simulink model "proj7_highway"  (R2016b)
settings: Solver=ode4  StartTime=0.0  StopTime=765  FixedStep=1  RelTol=1e-3  EnableMultiTasking=on
values from neighbouring files (symbols this model uses):
  V = sch_cycle(:,2)    [Motor_plot.m]
undefined symbols (not defined in the file or in its folder): mc
settings Model: Creator=dave0651  LastModifiedBy=Jinesh
settings OptimizationCC: LifeSpan=inf
settings DebuggingCC: SFUnexpectedBacktrackingDiag=warning  SFNoUnconditionalDefaultTransitionDiag=warning  SFExecutionAtInitializationDiag=none
settings GRTTargetCC: TargetLangStandard=C89/C90 (ANSI)  GeneratePreprocessorConditionals=Disable all
settings ConfigComp: CovMetricSettings=dw  CovHtmlReporting=on  CovSaveCumulativeToWorkspaceVar=on  CovSaveSingleToWorkspaceVar=on  CovExternalEMLEnable=off

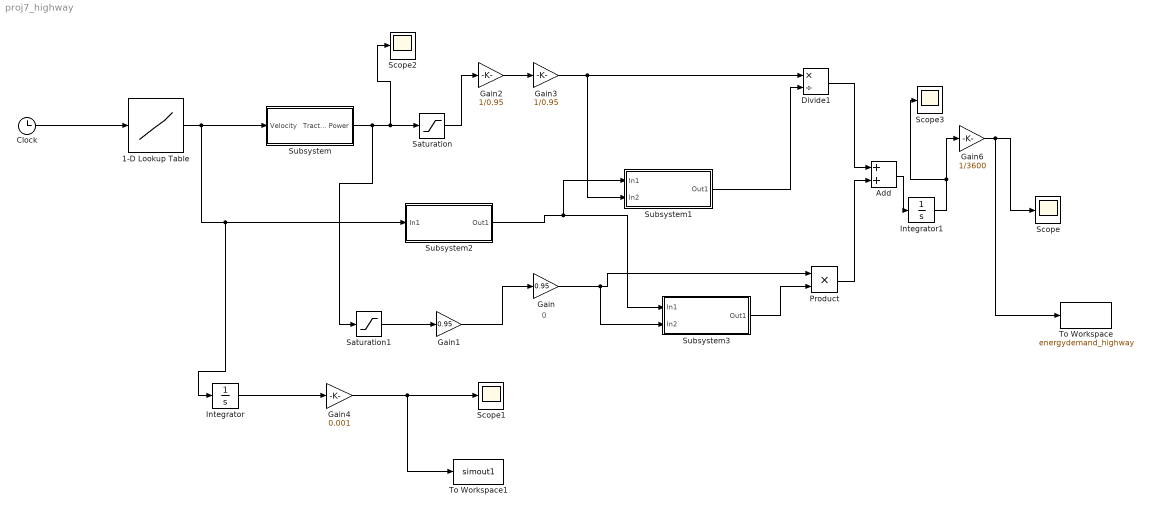
== system proj7_highway ==
  note: 0
  1-D Lookup Table : Lookup_n-D  NumberOfTableDimensions=1  BreakpointsForDimension1=t  Table=V  InternalRulePriority=Speed  RndMeth=Simplest  InputSameDT=on
  Add : Sum
  Clock : Clock
  Divide1 : Product  Inputs=*/
  Gain : Gain  Gain=0.95
  Gain1 : Gain  Gain=0.95
  Gain2 : Gain  Gain=1/0.95
  Gain3 : Gain  Gain=1/0.95
  Gain4 : Gain  Gain=0.001
  Gain6 : Gain  Gain=1/3600
  Integrator : Integrator
  Integrator1 : Integrator
  Product : Product
  Saturation : Saturate  UpperLimit=inf  LowerLimit=0
  Saturation1 : Saturate  UpperLimit=0  LowerLimit=-inf
  Scope{,1..3} (4 alike) : Scope
  Subsystem : Subsystem
  Subsystem1 : Subsystem
  Subsystem2 : Subsystem
  Subsystem3 : Subsystem
  To Workspace : ToWorkspace  VariableName=energydemand_highway  SaveFormat=Timeseries  SampleTime=-1
  To Workspace1 : ToWorkspace  VariableName=simout1  SaveFormat=Timeseries  SampleTime=-1
  wires:
  Clock/1 -> 1-D Lookup Table/1
  Saturation/1 -> Gain2/1
  Gain3/1 -> Subsystem1/2(In2), Divide1/1
  Subsystem2/1(Out1) -> Subsystem1/1(In1), Subsystem3/1(In1)
  Subsystem1/1(Out1) -> Divide1/2
  Add/1 -> Integrator1/1
  Product/1 -> Add/2
  Subsystem3/1(Out1) -> Product/2
  Gain1/1 -> Gain/1
  Saturation1/1 -> Gain1/1
  Gain/1 -> Subsystem3/2(In2), Product/1
  Gain4/1 -> To Workspace1/1, Scope1/1
  Integrator/1 -> Gain4/1
  Subsystem/1(Tractive Power) -> Saturation1/1, Scope2/1, Saturation/1
  1-D Lookup Table/1 -> Subsystem/1(Velocity), Integrator/1, Subsystem2/1(In1)
  Integrator1/1 -> Scope3/1, Gain6/1
  Gain6/1 -> To Workspace/1, Scope/1
  Gain2/1 -> Gain3/1
  Divide1/1 -> Add/1

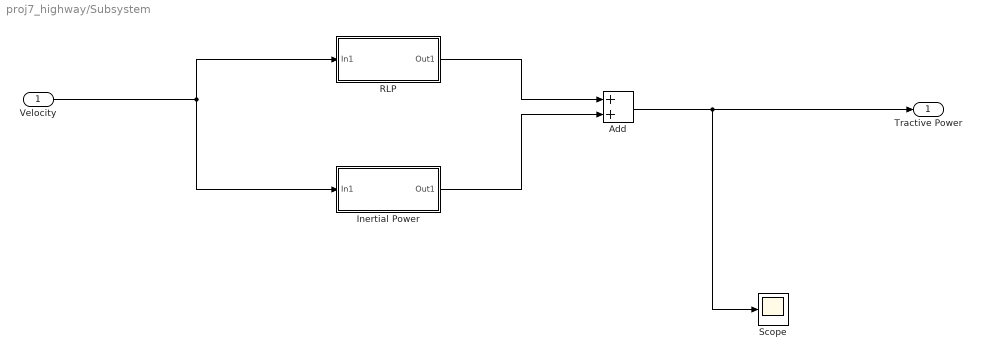
== system proj7_highway/Subsystem ==
  Velocity : Inport
  Add : Sum
  Inertial Power : Subsystem
  RLP : Subsystem
  Scope : Scope
  Tractive Power : Outport
  wires:
  Velocity/1 -> Inertial Power/1(In1), RLP/1(In1)
  Inertial Power/1(Out1) -> Add/2
  RLP/1(Out1) -> Add/1
  Add/1 -> Scope/1, Tractive Power/1

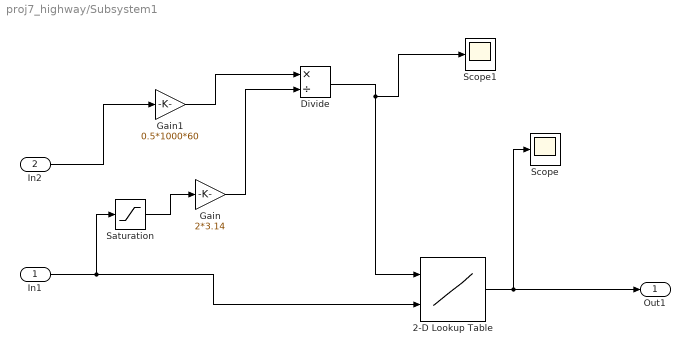
== system proj7_highway/Subsystem1 ==
  In1 : Inport
  In2 : Inport  Port=2
  2-D Lookup Table : Lookup_n-D  BreakpointsForDimension1=mc.trq_eff_index  BreakpointsForDimension2=mc.rpm_eff_index  Table=mc.eff_trq_map'  InternalRulePriority=Speed  RndMeth=Simplest  InputSameDT=on
  Divide : Product  Inputs=*/
  Gain : Gain  Gain=2*3.14
  Gain1 : Gain  Gain=0.5*1000*60
  Saturation : Saturate  UpperLimit=8000  LowerLimit=0.1
  Scope : Scope
  Scope1 : Scope
  Out1 : Outport
  wires:
  Gain/1 -> Divide/2
  In2/1 -> Gain1/1
  Gain1/1 -> Divide/1
  2-D Lookup Table/1 -> Scope/1, Out1/1
  In1/1 -> Saturation/1, 2-D Lookup Table/2
  Saturation/1 -> Gain/1
  Divide/1 -> Scope1/1, 2-D Lookup Table/1

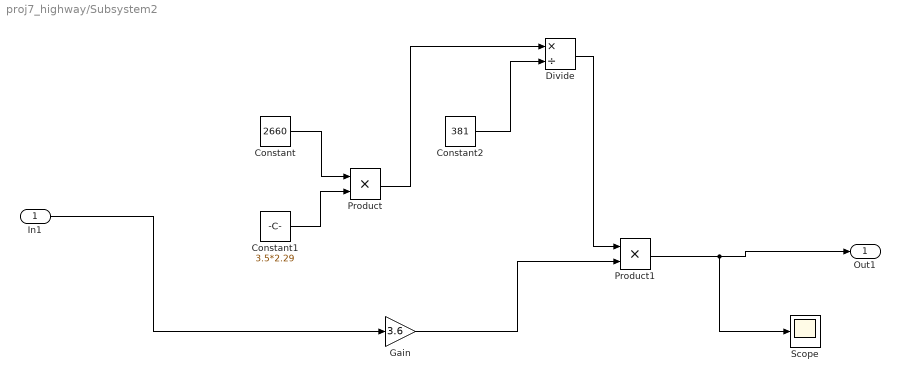
== system proj7_highway/Subsystem2 ==
  In1 : Inport
  Constant : Constant  Value=2660
  Constant1 : Constant  Value=3.5*2.29
  Constant2 : Constant  Value=381
  Divide : Product  Inputs=*/
  Gain : Gain  Gain=3.6
  Product : Product
  Product1 : Product
  Scope : Scope
  Out1 : Outport
  wires:
  Constant1/1 -> Product/2
  Constant/1 -> Product/1
  Product/1 -> Divide/1
  Divide/1 -> Product1/1
  Product1/1 -> Scope/1, Out1/1
  In1/1 -> Gain/1
  Gain/1 -> Product1/2
  Constant2/1 -> Divide/2

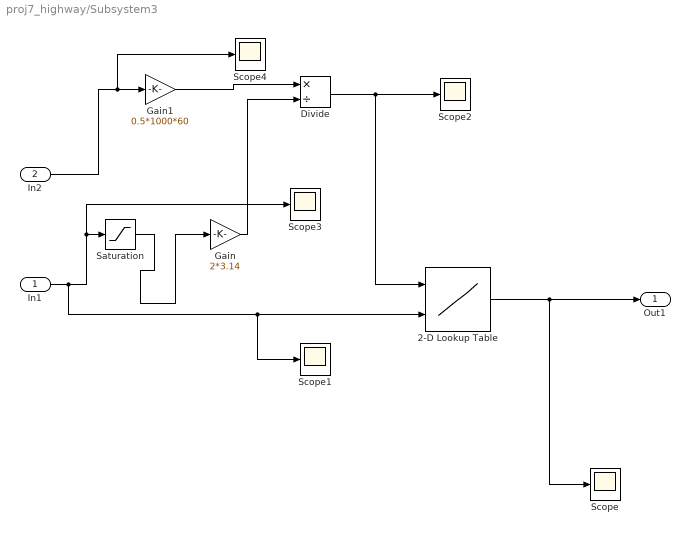
== system proj7_highway/Subsystem3 ==
  In1 : Inport
  In2 : Inport  Port=2
  2-D Lookup Table : Lookup_n-D  BreakpointsForDimension1=mc.trq_eff_index_gen  BreakpointsForDimension2=mc.rpm_eff_index_gen  Table=mc.eff_trq_map_gen'  InternalRulePriority=Speed  RndMeth=Simplest  InputSameDT=on
  Divide : Product  Inputs=*/
  Gain : Gain  Gain=2*3.14
  Gain1 : Gain  Gain=0.5*1000*60
  Saturation : Saturate  UpperLimit=8000  LowerLimit=0.1
  Scope{,1..4} (5 alike) : Scope
  Out1 : Outport
  wires:
  In1/1 -> Scope1/1, 2-D Lookup Table/2, Scope3/1, Saturation/1
  Saturation/1 -> Gain/1
  In2/1 -> Scope4/1, Gain1/1
  2-D Lookup Table/1 -> Scope/1, Out1/1
  Divide/1 -> Scope2/1, 2-D Lookup Table/1
  Gain/1 -> Divide/2
  Gain1/1 -> Divide/1

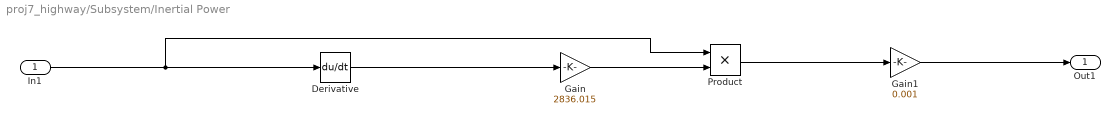
== system proj7_highway/Subsystem/Inertial Power ==
  In1 : Inport
  Derivative : Derivative
  Gain : Gain  Gain=2836.015
  Gain1 : Gain  Gain=0.001
  Product : Product
  Out1 : Outport
  wires:
  In1/1 -> Product/1, Derivative/1
  Derivative/1 -> Gain/1
  Gain/1 -> Product/2
  Product/1 -> Gain1/1
  Gain1/1 -> Out1/1

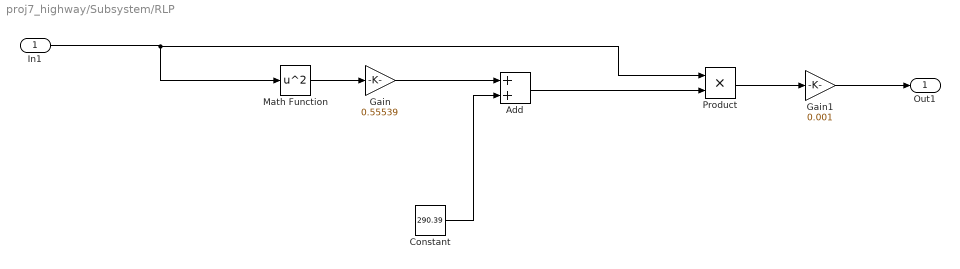
== system proj7_highway/Subsystem/RLP ==
  In1 : Inport
  Add : Sum
  Constant : Constant  Value=290.39
  Gain : Gain  Gain=0.55539
  Gain1 : Gain  Gain=0.001
  Math Function : Math  Operator=square  SaturateOnIntegerOverflow=on
  Product : Product
  Out1 : Outport
  wires:
  In1/1 -> Product/1, Math Function/1
  Math Function/1 -> Gain/1
  Gain/1 -> Add/1
  Constant/1 -> Add/2
  Add/1 -> Product/2
  Product/1 -> Gain1/1
  Gain1/1 -> Out1/1
